simulink model "HalfCar_Model"  (R2018b)
settings: Solver=VariableStepAuto  StartTime=0.0  StopTime=15  RelTol=1e-3
values from neighbouring files (symbols this model uses):
  a = 1.25    [SetCoefficients.m]    (also in SetCoefficients_HC.m)
  amplitude = 0.01    [SetCoefficients.m]    (also in SetCoefficients_HC.m)
  b = 1.4    [SetCoefficients.m]    (also in SetCoefficients_HC.m)
  csc = 600    [SetCoefficients.m]    (also in SetCoefficients_HC.m)
  cse = 1200    [SetCoefficients.m]    (also in SetCoefficients_HC.m)
  delay = (a+b)/v    (= 2.65)    [SetCoefficients.m]    (also in SetCoefficients_HC.m)
  Fre_r = Fre*2*pi    [SetCoefficients.m]    (also in SetCoefficients_HC.m)
  g = 9.81    [SetCoefficients.m]    (also in SetCoefficients_HC.m)
  I = 600    [SetCoefficients.m]    (also in SetCoefficients_HC.m)
  ks = 2e4    (= 20000)    [SetCoefficients.m]    (also in SetCoefficients_HC.m)
  ksstiff = 20*ks    (= 400000)    [SetCoefficients.m]    (also in SetCoefficients_HC.m)
  kt = 14e4    (= 140000)    [SetCoefficients.m]    (also in SetCoefficients_HC.m)
  m2 = 20    [SetCoefficients.m]    (also in SetCoefficients_HC.m)
  mb = 500    [SetCoefficients.m]    (also in SetCoefficients_HC.m)
  x1 = 0.2    [SetCoefficients.m]    (also in SetCoefficients_HC.m)
  x2 = 0.5    [SetCoefficients.m]    (also in SetCoefficients_HC.m)
settings Model: Creator=joebe  LastModifiedBy=joebe

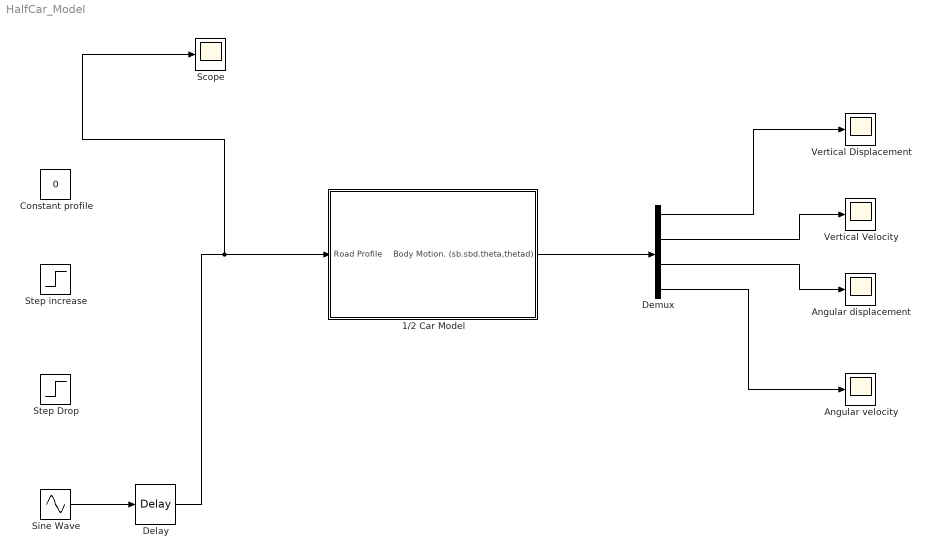
== system HalfCar_Model ==
  1/2 Car Model : Subsystem
  Angular displacement : Scope
  Angular velocity : Scope
  Constant profile : Constant  Value=0
  Delay : TransportDelay  DelayTime=5  BufferSize=3072
  Demux : Demux
  Scope : Scope
  Sine Wave : Sin  Amplitude=amplitude  Frequency=Fre_r  SampleTime=0
  Step Drop : Step  Time=2  After=-2  SampleTime=0
  Step increase : Step  Time=2  SampleTime=0
  Vertical Displacement : Scope
  Vertical Velocity : Scope
  wires:
  1/2 Car Model/1(Body Motion. (sb.sbd.theta,thetad)) -> Demux/1
  Demux/1 -> Vertical Displacement/1
  Demux/2 -> Vertical Velocity/1
  Demux/3 -> Angular displacement/1
  Demux/4 -> Angular velocity/1
  Sine Wave/1 -> Delay/1
  Delay/1 -> Scope/1, 1/2 Car Model/1(Road Profile)

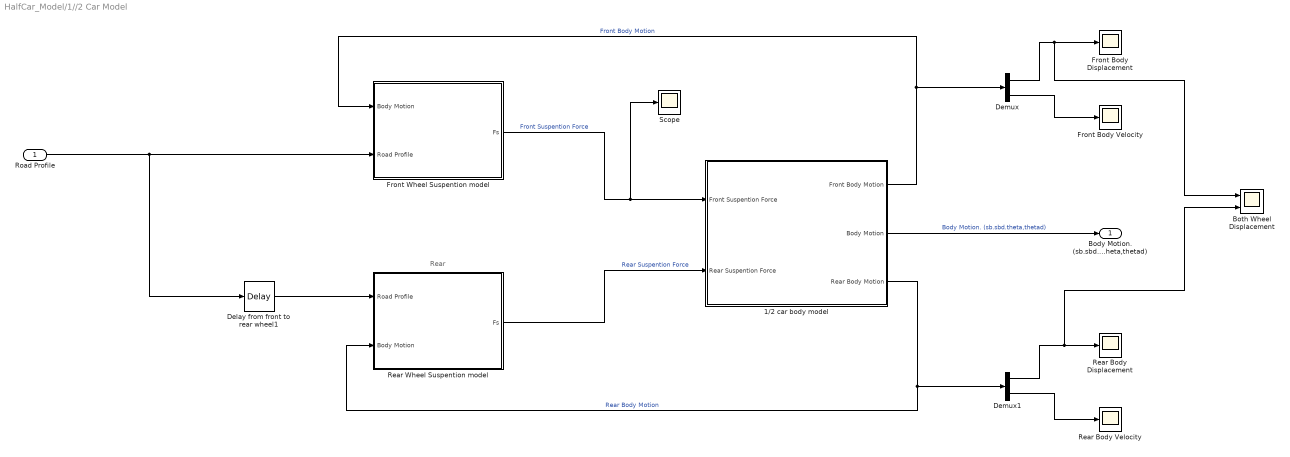
== system HalfCar_Model/1//2 Car Model ==
  note: Rear
  Road Profile : Inport
  1/2 car body model : Subsystem
  Both Wheel Displacement : Scope  NumInputPorts=2
  Delay from front to rear wheel1 : TransportDelay  DelayTime=delay  BufferSize=3072
  Demux : Demux  Outputs=2
  Demux1 : Demux  Outputs=2
  Front Body Displacement : Scope
  Front Body Velocity : Scope
  Front Wheel Suspention model : Subsystem
  Rear Body Displacement : Scope
  Rear Body Velocity : Scope
  Rear Wheel Suspention model : Subsystem
  Scope : Scope
  Body Motion. (sb.sbd.theta,thetad) : Outport
  wires:
  1/2 car body model/3(Rear Body Motion) -> Demux1/1, Rear Wheel Suspention model/2(Body Motion)  "Rear Body Motion"
  Demux1/2 -> Rear Body Velocity/1
  Demux/2 -> Front Body Velocity/1
  Road Profile/1 -> Delay from front to rear wheel1/1, Front Wheel Suspention model/2(Road Profile)
  Demux/1 -> Both Wheel Displacement/1, Front Body Displacement/1
  Demux1/1 -> Both Wheel Displacement/2, Rear Body Displacement/1
  Front Wheel Suspention model/1(Fs) -> Scope/1, 1/2 car body model/1(Front Suspention Force)  "Front Suspention Force"
  Rear Wheel Suspention model/1(Fs) -> 1/2 car body model/2(Rear Suspention Force)  "Rear Suspention Force"
  1/2 car body model/1(Front Body Motion) -> Demux/1, Front Wheel Suspention model/1(Body Motion)  "Front Body Motion"
  1/2 car body model/2(Body Motion) -> Body Motion. (sb.sbd.theta,thetad)/1  "Body Motion. (sb.sbd.theta,thetad)"
  Delay from front to rear wheel1/1 -> Rear Wheel Suspention model/1(Road Profile)

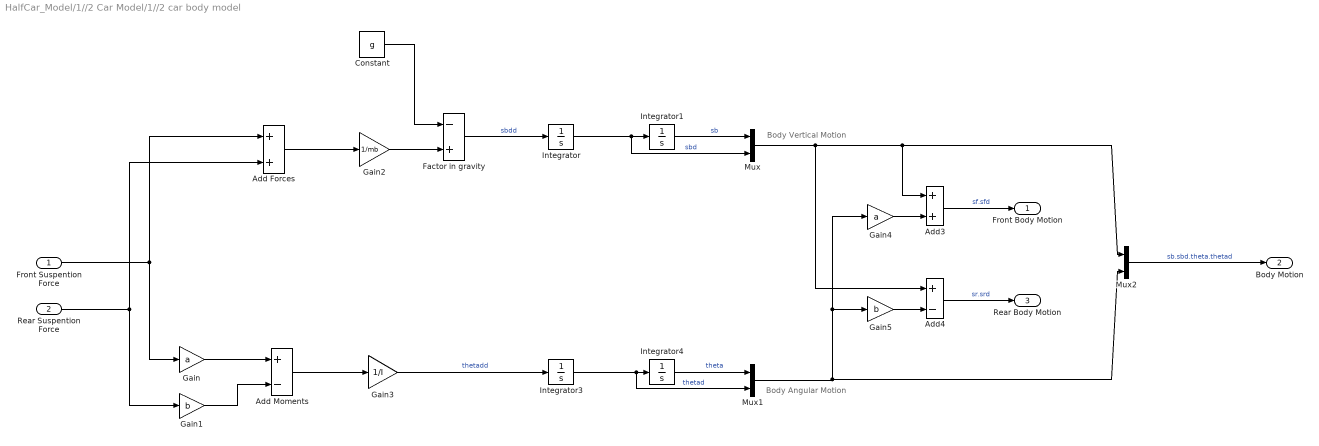
== system HalfCar_Model/1//2 Car Model/1//2 car body model ==
  note: Body Angular Motion
  note: Body Vertical Motion
  Front Suspention Force : Inport
  Rear Suspention Force : Inport  Port=2
  Add Forces : Sum
  Add Moments : Sum  Inputs=+-
  Add3 : Sum
  Add4 : Sum  Inputs=+-
  Constant : Constant  Value=g
  Factor in gravity : Sum  Inputs=-+
  Gain : Gain  Gain=a
  Gain1 : Gain  Gain=b
  Gain2 : Gain  Gain=1/mb
  Gain3 : Gain  Gain=1/I
  Gain4 : Gain  Gain=a
  Gain5 : Gain  Gain=b
  Integrator{,1,3..4} (4 alike) : Integrator
  Mux : Mux  Inputs=2
  Mux1 : Mux  Inputs=2
  Mux2 : Mux  Inputs=2
  Front Body Motion : Outport
  Body Motion : Outport  Port=2
  Rear Body Motion : Outport  Port=3
  wires:
  Add Forces/1 -> Gain2/1
  Mux1/1 -> Gain4/1, Gain5/1, Mux2/2
  Integrator3/1 -> Mux1/2, Integrator4/1  "thetad"
  Add Moments/1 -> Gain3/1
  Gain3/1 -> Integrator3/1  "thetadd"
  Mux2/1 -> Body Motion/1  "sb.sbd.theta.thetad"
  Gain2/1 -> Factor in gravity/2
  Mux/1 -> Add4/1, Add3/1, Mux2/1
  Gain4/1 -> Add3/2
  Gain/1 -> Add Moments/1
  Integrator4/1 -> Mux1/1  "theta"
  Integrator/1 -> Mux/2, Integrator1/1  "sbd"
  Rear Suspention Force/1 -> Add Forces/2, Gain1/1
  Front Suspention Force/1 -> Gain/1, Add Forces/1
  Integrator1/1 -> Mux/1  "sb"
  Gain1/1 -> Add Moments/2
  Add3/1 -> Front Body Motion/1  "sf.sfd"
  Gain5/1 -> Add4/2
  Constant/1 -> Factor in gravity/1
  Factor in gravity/1 -> Integrator/1  "sbdd"
  Add4/1 -> Rear Body Motion/1  "sr.srd"

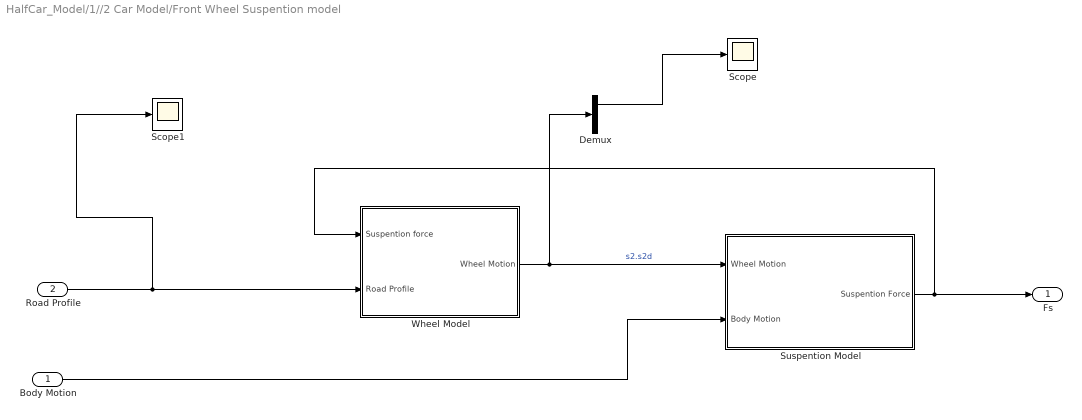
== system HalfCar_Model/1//2 Car Model/Front Wheel Suspention model ==
  Body Motion : Inport
  Road Profile : Inport  Port=2
  Demux : Demux  Outputs=2
  Scope : Scope
  Scope1 : Scope
  Suspention Model : Subsystem
  Wheel Model : Subsystem
  Fs : Outport
  wires:
  Wheel Model/1(Wheel Motion) -> Demux/1, Suspention Model/1(Wheel Motion)  "s2.s2d"
  Road Profile/1 -> Scope1/1, Wheel Model/2(Road Profile)
  Suspention Model/1(Suspention Force) -> Fs/1, Wheel Model/1(Suspention force)
  Body Motion/1 -> Suspention Model/2(Body Motion)
  Demux/1 -> Scope/1

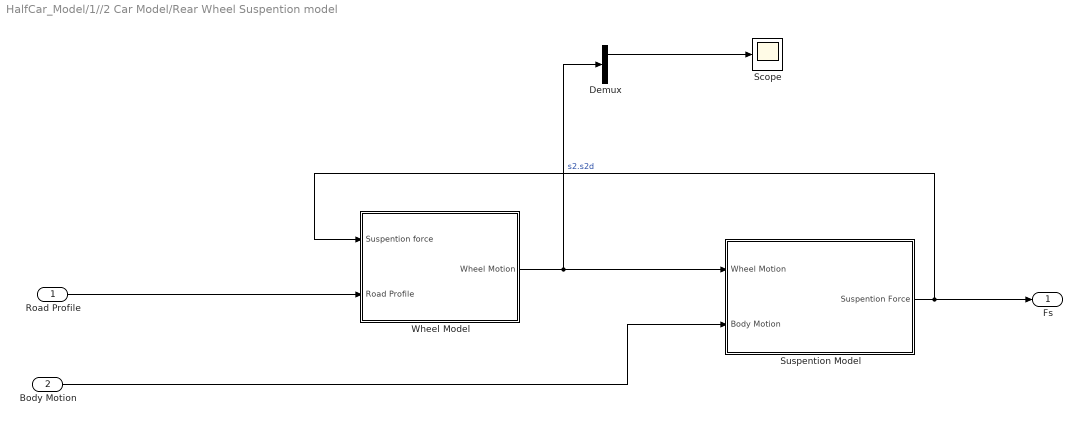
== system HalfCar_Model/1//2 Car Model/Rear Wheel Suspention model ==
  Road Profile : Inport
  Body Motion : Inport  Port=2
  Demux : Demux  Outputs=2
  Scope : Scope
  Suspention Model : Subsystem
  Wheel Model : Subsystem
  Fs : Outport
  wires:
  Wheel Model/1(Wheel Motion) -> Demux/1, Suspention Model/1(Wheel Motion)  "s2.s2d"
  Road Profile/1 -> Wheel Model/2(Road Profile)
  Suspention Model/1(Suspention Force) -> Fs/1, Wheel Model/1(Suspention force)
  Body Motion/1 -> Suspention Model/2(Body Motion)
  Demux/1 -> Scope/1

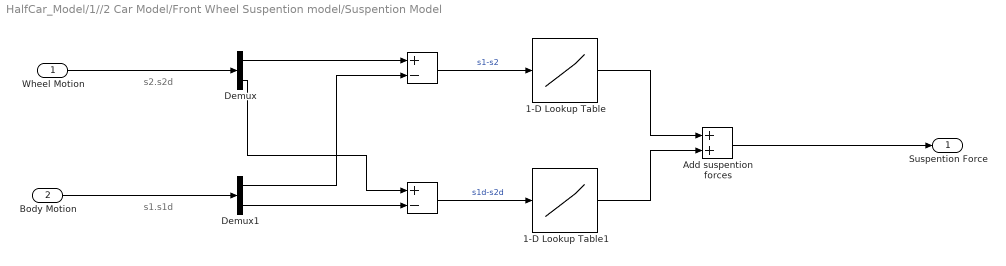
== system HalfCar_Model/1//2 Car Model/Front Wheel Suspention model/Suspention Model ==
  note: s1.s1d
  note: s2.s2d
  Wheel Motion : Inport
  Body Motion : Inport  Port=2
  " " : Sum  Inputs=+-
  " " : Sum  Inputs=+-
  1-D Lookup Table : Lookup_n-D  NumberOfTableDimensions=1  BreakpointsForDimension1=[-x2 -x1 x1 x2]  Table=[-(ksstiff*(x2-x1)+ks*x1) -x1*ks x1*ks (ksstiff*(x2-x1)+ks*x1)]  InternalRulePriority=Speed  RndMeth=Simplest  InputSameDT=on
  1-D Lookup Table1 : Lookup_n-D  NumberOfTableDimensions=1  BreakpointsForDimension1=[-10 0 10]  Table=[-10*cse 0 10*csc]  InternalRulePriority=Speed  RndMeth=Simplest  InputSameDT=on
  Add suspention forces : Sum
  Demux : Demux  Outputs=2
  Demux1 : Demux  Outputs=2
  Suspention Force : Outport
  wires:
  Demux1/2 -> " "/2
  " "/1 -> 1-D Lookup Table/1  "s1-s2"
  Demux1/1 -> " "/2
  1-D Lookup Table1/1 -> Add suspention forces/2
  1-D Lookup Table/1 -> Add suspention forces/1
  Demux/1 -> " "/1
  Demux/2 -> " "/1
  Body Motion/1 -> Demux1/1
  " "/1 -> 1-D Lookup Table1/1  "s1d-s2d"
  Add suspention forces/1 -> Suspention Force/1
  Wheel Motion/1 -> Demux/1

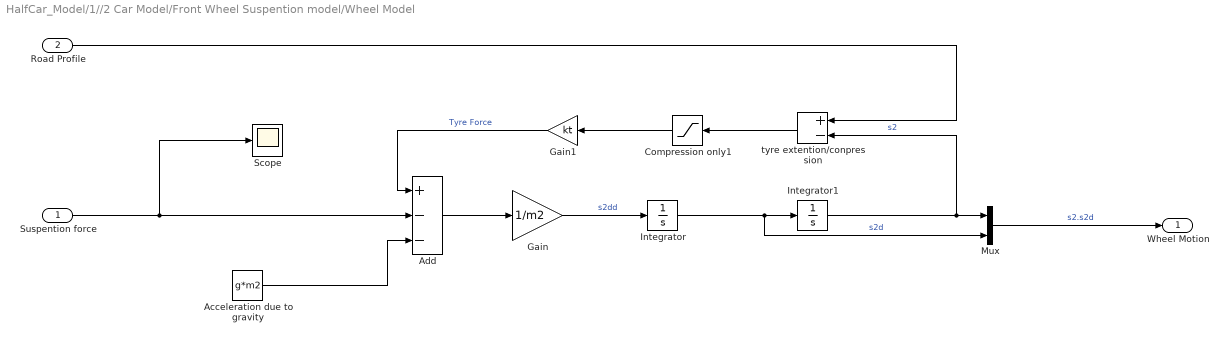
== system HalfCar_Model/1//2 Car Model/Front Wheel Suspention model/Wheel Model ==
  Suspention force : Inport
  Road Profile : Inport  Port=2
  Acceleration due to gravity : Constant  Value=g*m2
  Add : Sum  Inputs=+--
  Compression only1 : Saturate  UpperLimit=inf  LowerLimit=0
  Gain : Gain  Gain=1/m2
  Gain1 : Gain  Gain=kt
  Integrator : Integrator
  Integrator1 : Integrator
  Mux : Mux  Inputs=2
  Scope : Scope
  tyre extention/conpression : Sum  Inputs=+-
  Wheel Motion : Outport
  wires:
  Integrator1/1 -> Mux/1, tyre extention/conpression/2  "s2"
  Integrator/1 -> Mux/2, Integrator1/1  "s2d"
  Add/1 -> Gain/1
  Gain1/1 -> Add/1  "Tyre Force"
  Road Profile/1 -> tyre extention/conpression/1
  Mux/1 -> Wheel Motion/1  "s2.s2d"
  Acceleration due to gravity/1 -> Add/3
  Suspention force/1 -> Scope/1, Add/2
  Gain/1 -> Integrator/1  "s2dd"
  tyre extention/conpression/1 -> Compression only1/1
  Compression only1/1 -> Gain1/1

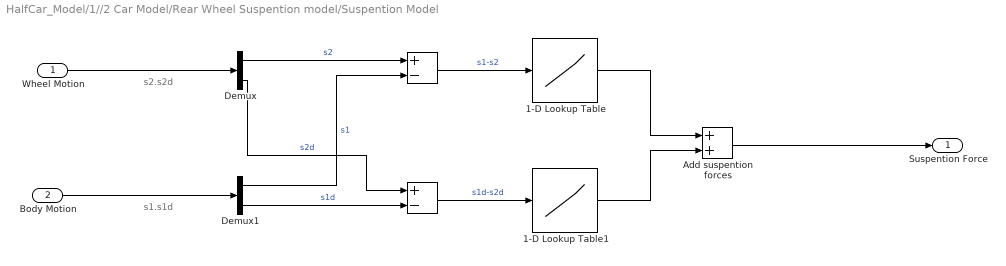
== system HalfCar_Model/1//2 Car Model/Rear Wheel Suspention model/Suspention Model ==
  note: s1.s1d
  note: s2.s2d
  Wheel Motion : Inport
  Body Motion : Inport  Port=2
  " " : Sum  Inputs=+-
  " " : Sum  Inputs=+-
  1-D Lookup Table : Lookup_n-D  NumberOfTableDimensions=1  BreakpointsForDimension1=[-x2 -x1 x1 x2]  Table=[-(ksstiff*(x2-x1)+ks*x1) -x1*ks x1*ks (ksstiff*(x2-x1)+ks*x1)]  InternalRulePriority=Speed  RndMeth=Simplest  InputSameDT=on
  1-D Lookup Table1 : Lookup_n-D  NumberOfTableDimensions=1  BreakpointsForDimension1=[-10 0 10]  Table=[-10*cse 0 10*csc]  InternalRulePriority=Speed  RndMeth=Simplest  InputSameDT=on
  Add suspention forces : Sum
  Demux : Demux  Outputs=2
  Demux1 : Demux  Outputs=2
  Suspention Force : Outport
  wires:
  Demux1/2 -> " "/2  "s1d"
  " "/1 -> 1-D Lookup Table/1  "s1-s2"
  Demux1/1 -> " "/2  "s1"
  1-D Lookup Table1/1 -> Add suspention forces/2
  1-D Lookup Table/1 -> Add suspention forces/1
  Demux/1 -> " "/1  "s2"
  Demux/2 -> " "/1  "s2d"
  Body Motion/1 -> Demux1/1
  " "/1 -> 1-D Lookup Table1/1  "s1d-s2d"
  Add suspention forces/1 -> Suspention Force/1
  Wheel Motion/1 -> Demux/1

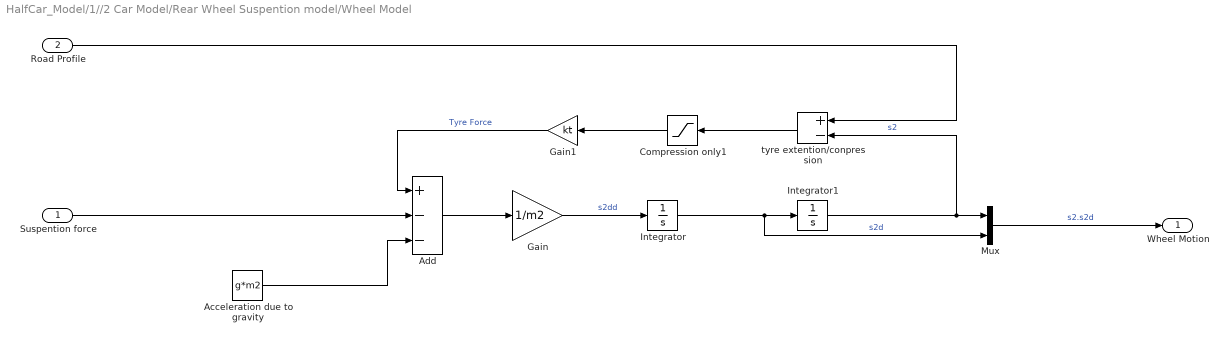
== system HalfCar_Model/1//2 Car Model/Rear Wheel Suspention model/Wheel Model ==
  Suspention force : Inport
  Road Profile : Inport  Port=2
  Acceleration due to gravity : Constant  Value=g*m2
  Add : Sum  Inputs=+--
  Compression only1 : Saturate  UpperLimit=inf  LowerLimit=0
  Gain : Gain  Gain=1/m2
  Gain1 : Gain  Gain=kt
  Integrator : Integrator
  Integrator1 : Integrator
  Mux : Mux  Inputs=2
  tyre extention/conpression : Sum  Inputs=+-
  Wheel Motion : Outport
  wires:
  Integrator1/1 -> tyre extention/conpression/2, Mux/1  "s2"
  Integrator/1 -> Mux/2, Integrator1/1  "s2d"
  Add/1 -> Gain/1
  Gain1/1 -> Add/1  "Tyre Force"
  Road Profile/1 -> tyre extention/conpression/1
  Mux/1 -> Wheel Motion/1  "s2.s2d"
  Acceleration due to gravity/1 -> Add/3
  Suspention force/1 -> Add/2
  Gain/1 -> Integrator/1  "s2dd"
  tyre extention/conpression/1 -> Compression only1/1
  Compression only1/1 -> Gain1/1
